simulink model "Animation"  (R2023b)
settings: Solver=VariableStepAuto  StartTime=0.0  StopTime=200  RelTol=1e-3
libraries: uavutilslib x2, robotcorelib x1
settings Model: Creator=DELL  LastModifiedBy=DELL

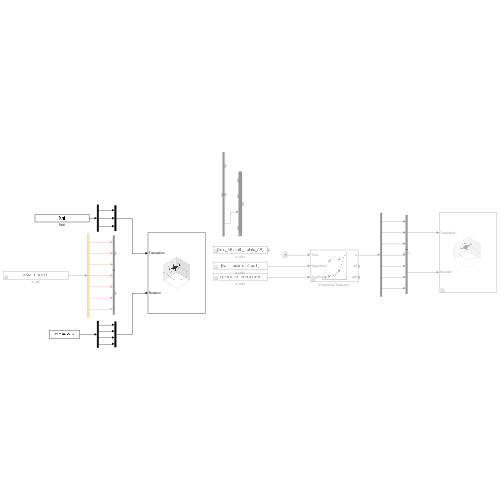
[thumbnail: Simulink's stored preview of the top-level diagram]
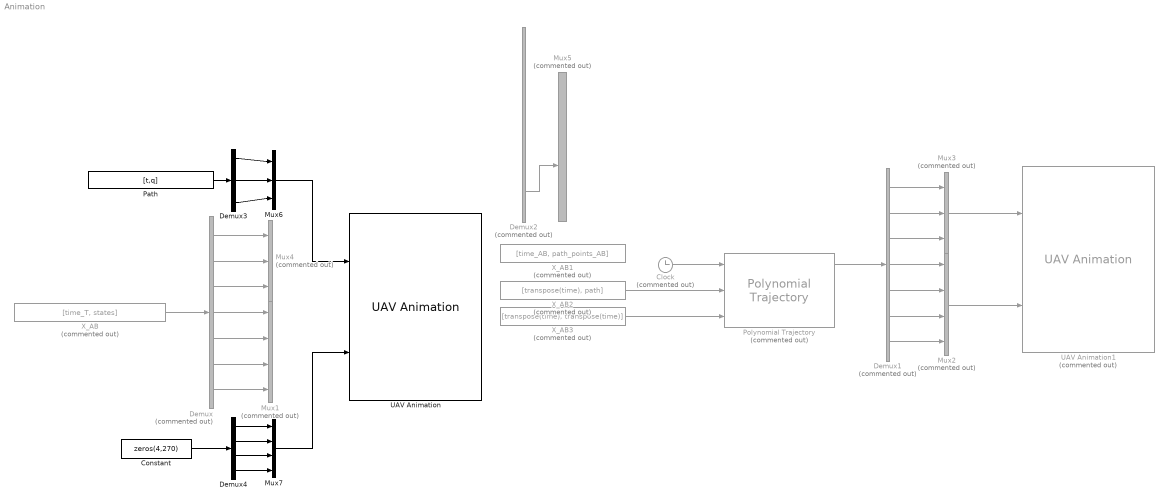
== system Animation ==
  Clock : Clock  Commented=on
  Constant : Constant  Value=zeros(4,270)
  Demux : Demux  Commented=on  Outputs=7
  Demux1 : Demux  Commented=on  Outputs=7
  Demux2 : Demux  Commented=on  Outputs=3
  Demux3 : Demux  Outputs=3
  Demux4 : Demux
  Mux1 : Mux  Commented=on
  Mux2 : Mux  Commented=on
  Mux3 : Mux  Commented=on  Inputs=3
  Mux4 : Mux  Commented=on  Inputs=3
  Mux5 : Mux  Commented=on
  Mux6 : Mux  Inputs=3
  Mux7 : Mux
  Path : FromWorkspace  VariableName=[t,q]
  Polynomial Trajectory : robotcorelib/Polynomial Trajectory  Commented=on  WaypointSource=External  Waypoints=[ 0, 2, 1, 5, 0; -1, 3, 1, 4, 4 ]  TimePoints=[ 0, 1, 2, 3, 4 ]  TimeInterval=[ 1, 4 ]  Method=Quintic Polynomial  ParameterSource=Internal  VelocityBoundaryCondition=zeros( 2, 5 )  AccelerationBoundaryCondition=zeros( 2, 5 )  SimulateUsing=Interpreted execution
  UAV Animation : uavutilslib/UAV Animation  UAVType=Multirotor  UAVSize=1  InertialZDirection=Up  SampleTime=-1
  UAV Animation1 : uavutilslib/UAV Animation  Commented=on  UAVType=Multirotor  UAVSize=1  InertialZDirection=Up  SampleTime=-1
  X_AB : FromWorkspace  Commented=on  VariableName=[time_T, states]
  X_AB1 : FromWorkspace  Commented=on  VariableName=[time_AB, path_points_AB]
  X_AB2 : FromWorkspace  Commented=on  VariableName=[transpose(time), path]
  X_AB3 : FromWorkspace  Commented=on  VariableName=[transpose(time), transpose(time)]
  wires:
  Demux/1 -> Mux4/1
  Demux/2 -> Mux4/2
  Demux/3 -> Mux4/3
  Demux/4 -> Mux1/1
  Demux/5 -> Mux1/2
  Demux/6 -> Mux1/3
  Demux/7 -> Mux1/4
  Demux1/2 -> Mux3/2
  Demux1/7 -> Mux2/4
  Polynomial Trajectory/1 -> Demux1/1
  Demux1/4 -> Mux2/1
  Mux2/1 -> UAV Animation1/2
  Demux1/3 -> Mux3/3
  Demux1/1 -> Mux3/1
  Mux3/1 -> UAV Animation1/1
  Demux1/6 -> Mux2/3
  Demux1/5 -> Mux2/2
  X_AB2/1 -> Polynomial Trajectory/2
  Clock/1 -> Polynomial Trajectory/1
  Demux2/3 -> Mux5/3
  X_AB3/1 -> Polynomial Trajectory/3
  X_AB/1 -> Demux/1
  Demux3/2 -> Mux6/2
  Demux3/1 -> Mux6/1
  Demux3/3 -> Mux6/3
  Path/1 -> Demux3/1
  Mux6/1 -> UAV Animation/1
  Demux4/1 -> Mux7/1
  Demux4/2 -> Mux7/2
  Demux4/3 -> Mux7/3
  Demux4/4 -> Mux7/4
  Constant/1 -> Demux4/1
  Mux7/1 -> UAV Animation/2
